simulink model "B_3_13"  (R2016b)
settings: Solver=VariableStepAuto  StartTime=0.0  StopTime=10.0  RelTol=1e-3
values from neighbouring files (symbols this model uses):
  b = 1    [hw5.m]    (also in hw5p1.m; hw5p1b.m = 10; hw5p1c.m = 0; hw5p1d.m = (2*sqrt(J*k)))
  J = 1    [hw5.m]    (also in hw5p1.m; hw5p1b.m; hw5p1c.m; hw5p1d.m)
  k = 10    [hw5.m]    (also in hw5p1.m; hw5p1b.m; hw5p1c.m; hw5p1d.m)
settings Model: Creator=Simon  LastModifiedBy=Simon

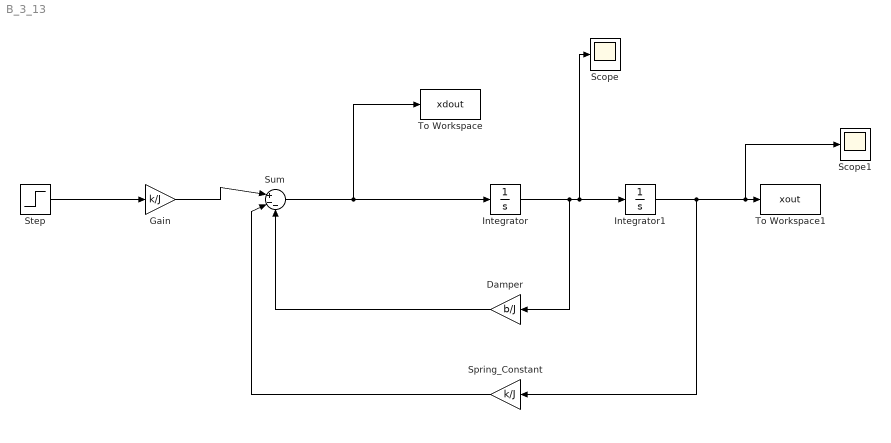
== system B_3_13 ==
  Damper : Gain  Gain=b/J
  Gain : Gain  Gain=k/J
  Integrator : Integrator
  Integrator1 : Integrator  InitialCondition=-1
  Scope : Scope
  Scope1 : Scope
  Spring_Constant : Gain  Gain=k/J
  Step : Step  Time=0  SampleTime=0
  Sum : Sum  Inputs=|+--
  To Workspace : ToWorkspace  VariableName=xdout  SaveFormat=Timeseries  SampleTime=-1
  To Workspace1 : ToWorkspace  VariableName=xout  SaveFormat=Timeseries  SampleTime=-1
  wires:
  Integrator/1 -> Damper/1, Scope/1, Integrator1/1
  Damper/1 -> Sum/3
  Spring_Constant/1 -> Sum/2
  Integrator1/1 -> Scope1/1, To Workspace1/1, Spring_Constant/1
  Step/1 -> Gain/1
  Gain/1 -> Sum/1
  Sum/1 -> To Workspace/1, Integrator/1
